simulink model "clik_transpose"  (R2022b)
settings: Solver=ode1  StartTime=0.0  StopTime=4  FixedStep=0.001  RelTol=1e-3
undefined symbols (not defined in the file or in its folder): DiscIntNeverNeededParam, q0, Tc
settings Model: Creator=Xp  LastModifiedBy=TAARUN
settings SolverCC: AlgebraicLoopSolver=TrustRegion
settings DataIOCC: LimitDataPoints=on  SaveFormat=Array  SignalLoggingSaveFormat=ModelDataLogs  ReturnWorkspaceOutputs=off
settings OptimizationCC: ExpressionDepthLimit=2147483647  InitFltsAndDblsToZero=on  LifeSpan=inf
settings DebuggingCC: SaveWithParameterizedLinksMsg=none  UnderspecifiedInitializationDetection=Classic  MergeDetectMultiDrivingBlocksExec=none  SolverPrmCheckMsg=warning  MultiTaskDSMMsg=warning  MultiTaskCondExecSysMsg=none  FcnCallInpInsideContextMsg=warning  UnconnectedInputMsg=warning  UnconnectedOutputMsg=warning  UnconnectedLineMsg=warning  StateNameClashWarn=warning  SFUnexpectedBacktrackingDiag=warning  SFNoUnconditionalDefaultTransitionDiag=warning  SFExecutionAtInitializationDiag=none  SFMachineParentedDataDiag=warning  ArithmeticOperatorsInVariantConditions=warning
settings HardwareCC: ProdBitPerPointer=32  ProdBitPerSizeT=32  ProdBitPerPtrDiffT=32  ProdLargestAtomicFloat=None  ProdIntDivRoundTo=Undefined  ProdEndianess=Unspecified  ProdWordSize=32  ProdHWDeviceType=32-bit Generic
settings ModelReferenceCC: EnableRefExpFcnMdlSchedulingChecks=on  PropagateSignalLabelsOutOfModel=off
settings SFSimCC: CustomCodeUndefinedFunction=UseInterfaceOnly
settings RTWCC: DLArmComputeVersion=19.05
settings CodeAppCC: StateflowObjectComments=on
settings GRTTargetCC: TargetLangStandard=C89/C90 (ANSI)  CombineOutputUpdateFcns=off  GRTInterface=on
settings ConfigComp: CovMetricSettings=dw  CovSaveCumulativeToWorkspaceVar=on  CovSaveSingleToWorkspaceVar=on

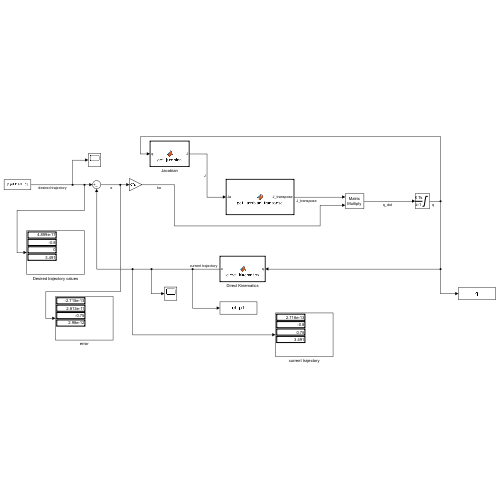
[thumbnail: Simulink's stored preview of the top-level diagram]
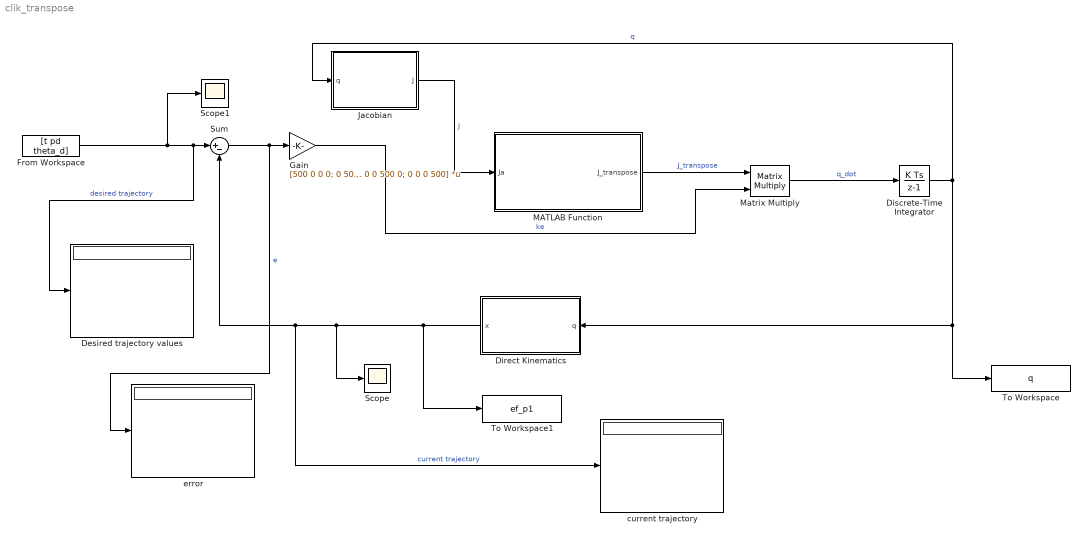
== system clik_transpose ==
  Desired trajectory values : Display
  Direct Kinematics : MATLAB Function  TreatAsAtomicUnit=on
  Discrete-Time Integrator : DiscreteIntegrator  InitialCondition=q0  SampleTime=Tc  LimitOutput=on  UpperSaturationLimit=[pi/2; pi/4; 1; 2*pi]  LowerSaturationLimit=[-pi/2; -pi/2; 0.25; -2*pi]  ICPrevOutput=DiscIntNeverNeededParam  ICPrevScaledInput=DiscIntNeverNeededParam
  From Workspace : FromWorkspace  VariableName=[t pd theta_d]  SampleTime=Tc
  Gain : Gain  Gain=[500 0 0 0; 0 500 0 0; 0 0 500 0; 0 0 0 500]  Multiplication=Matrix(K*u)
  Jacobian : MATLAB Function  TreatAsAtomicUnit=on
  MATLAB Function : MATLAB Function  TreatAsAtomicUnit=on
  Matrix Multiply : Product  Multiplication=Matrix(*)
  Scope : Scope
  Scope1 : Scope
  Sum : Sum  Inputs=|+-
  To Workspace : ToWorkspace  VariableName=q  SampleTime=Tc
  To Workspace1 : ToWorkspace  VariableName=ef_p1  SampleTime=Tc
  current trajectory : Display
  error : Display
  wires:
  From Workspace/1 -> Scope1/1, Desired trajectory values/1, Sum/1  "desired trajectory"
  Sum/1 -> error/1, Gain/1  "e"
  Jacobian/1(J) -> MATLAB Function/1(Ja)  "J"
  Discrete-Time Integrator/1 -> Jacobian/1(q), To Workspace/1, Direct Kinematics/1(q)  "q"
  Direct Kinematics/1(x) -> To Workspace1/1, Scope/1, current trajectory/1, Sum/2  "current trajectory"
  MATLAB Function/1(J_transpose) -> Matrix Multiply/1  "J_transpose"
  Gain/1 -> Matrix Multiply/2  "ke"
  Matrix Multiply/1 -> Discrete-Time Integrator/1  "q_dot"

== matlab function clik_transpose/Jacobian ==
  data: q input; J output
function J = get_jacobian(q)
    
J = jacobian(q);

== matlab function clik_transpose/Direct Kinematics ==
  data: q input; x output
function x = direct_kinematics(q)

x = direct_kin(q);

== matlab function clik_transpose/MATLAB Function ==
  data: Ja input; J_transpose output
function J_transpose = get_jacobian_transpose(Ja)

J_transpose = transpose(Ja);
